simulink model "ModeleSimulinkQ19"  (R2019b)
settings: Solver=VariableStepAuto  StartTime=0.0  StopTime=500  RelTol=1e-3
values from neighbouring files (symbols this model uses):
  qdf = [0 1 0 0 0 0]'    [TP2.m]
  qdi = [-1 0 -1 -1 -1 -1]'    [TP2.m]
settings Model: Creator=davide  LastModifiedBy=davide

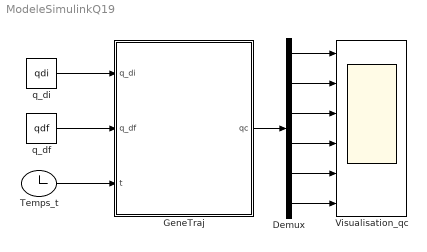
== system ModeleSimulinkQ19 ==
  Demux : Demux  Outputs=6
  GeneTraj : MATLAB Function  TreatAsAtomicUnit=on
  "Temps_t " : Clock
  Visualisation_qc : Scope  NumInputPorts=6
  "q_df " : Constant  Value=qdf  VectorParams1D=off
  q_di : Constant  Value=qdi  VectorParams1D=off
  wires:
  "q_df "/1 -> GeneTraj/2(q_df)
  "Temps_t "/1 -> GeneTraj/3(t)
  q_di/1 -> GeneTraj/1(q_di)
  Demux/6 -> Visualisation_qc/6
  GeneTraj/1(qc) -> Demux/1
  Demux/1 -> Visualisation_qc/1
  Demux/2 -> Visualisation_qc/2
  Demux/3 -> Visualisation_qc/3
  Demux/4 -> Visualisation_qc/4
  Demux/5 -> Visualisation_qc/5

== matlab function ModeleSimulinkQ19/GeneTraj ==
  data: q_di input; qc output; q_df input; t input
function qc = GeneTraj(q_di, q_df, t)
    
    tf = 500; %in ms
     
    D = (q_df - q_di);
    
    r = 10 * (t/tf)^3 - 15 * (t/tf)^4 + 6 * (t/tf)^5;
    
    qc = q_di + r*D;
end
